simulink model "DynMatProps"  (R2015a)
settings: Solver=FixedStepDiscrete  StartTime=0.0  StopTime=tsim  FixedStep=dt  RelTol=1e-3
values from neighbouring files (symbols this model uses):
  Cp_data = [4.8261 5.46958 6.4348 6.981758 7.56089 8.0435 8.68698]    [run_DynMatProps.m]
  hb = 0.05    [run_DynMatProps.m]
  hl = 0.05    [run_DynMatProps.m]
  hr = 0.05    [run_DynMatProps.m]
  ht = 0.05    [run_DynMatProps.m]
  k_data = [0.013888889 0.016388889 0.020277778 0.022222222 0.027777778 0.029166667 0.027777778]    [run_DynMatProps.m]
  m = length(y0)    [run_DynMatProps.m]
  n = length(x)    [run_DynMatProps.m]
  rho2d = rho*ones(length(y0),length(x))    [run_DynMatProps.m]
  T02d = [T02d T01d']    [run_DynMatProps.m]
  Tb = 1000    [run_DynMatProps.m]
  TCp_data = [259.7 359.7 559.7 659.7 859.7 1059.7 1259.7]    [run_DynMatProps.m]
  Tk_data = [259.7 359.7 559.7 659.7 859.7 1059.7 1259.7]    [run_DynMatProps.m]
  Tl = 1000    [run_DynMatProps.m]
  Tr = 1000    [run_DynMatProps.m]
  Tt = 1000    [run_DynMatProps.m]
libraries: lib_Conduction_2DCondFullyImplicit x1
settings Model: Creator=jlkratz  LastModifiedBy=jlkratz

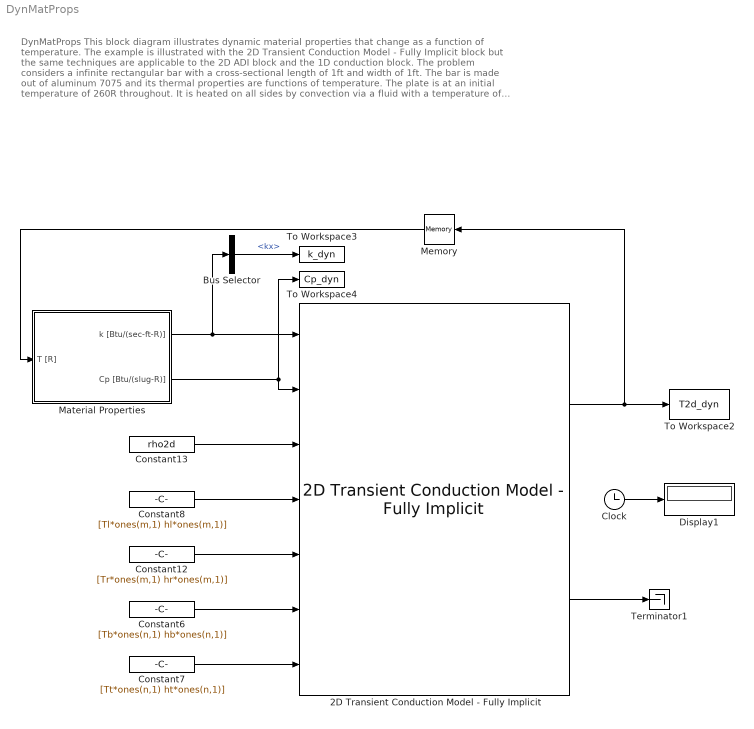
== system DynMatProps ==
  note: DynMatProps
      |
      | This block diagram illustrates dynamic material properties that change as a function of temperature. The example is
      | illustrated with the 2D Transient Conduction Model - Fully Implicit block but the same techniques are applicable
      | to the 2D ADI block and the 1D conduction block.
      |
      | The problem considers a infinite rectangular bar with a cross-sectional length of 1ft and width of 1ft. The bar is made
      | out of aluminum 7075 and its thermal properties are functions of temperature. The plate is at an initial temperature of
      | 260R throughout. It is heated on all sides by convection via a fluid with a temperature of 1000R and a heat transfer
      | coefficient of 0.05Btu/(sec-ft^2-R)
  2D Transient Conduction Model - Fully Implicit : lib_Conduction_2DCondFullyImplicit/2D Transient Conduction Model - Fully Implicit  T0_M=T02d  dt_M=dt  x_M=x  y_M=y0  shape_M=Planar in both directions  convL_M=on  radL_M=off  condL_M=off  convR_M=on  radR_M=off  condR_M=off  convB_M=on  radB_M=off  condB_M=off  convT_M=on  radT_M=off  condT_M=off  BN_M=double(gcb)
  Bus Selector : BusSelector  OutputSignals=kx
  Clock : Clock
  Constant12 : Constant  Value=[Tr*ones(m,1) hr*ones(m,1)]
  Constant13 : Constant  Value=rho2d
  Constant6 : Constant  Value=[Tb*ones(n,1) hb*ones(n,1)]
  Constant7 : Constant  Value=[Tt*ones(n,1) ht*ones(n,1)]
  Constant8 : Constant  Value=[Tl*ones(m,1) hl*ones(m,1)]
  Display1 : Display
  Material Properties : Subsystem
  Memory : Memory  X0=T02d
  Terminator1 : Terminator
  To Workspace2 : ToWorkspace  VariableName=T2d_dyn  SaveFormat=Timeseries  SampleTime=-1
  To Workspace3 : ToWorkspace  VariableName=k_dyn  SaveFormat=Timeseries  SampleTime=-1
  To Workspace4 : ToWorkspace  VariableName=Cp_dyn  SaveFormat=Timeseries  SampleTime=-1
  wires:
  Clock/1 -> Display1/1
  Constant7/1 -> 2D Transient Conduction Model - Fully Implicit/7
  Constant8/1 -> 2D Transient Conduction Model - Fully Implicit/4
  Constant12/1 -> 2D Transient Conduction Model - Fully Implicit/5
  Constant13/1 -> 2D Transient Conduction Model - Fully Implicit/3
  2D Transient Conduction Model - Fully Implicit/1 -> Memory/1, To Workspace2/1
  2D Transient Conduction Model - Fully Implicit/2 -> Terminator1/1
  Memory/1 -> Material Properties/1(T [R])
  Material Properties/1(k [Btu/(sec-ft-R)]) -> 2D Transient Conduction Model - Fully Implicit/1, Bus Selector/1
  Material Properties/2(Cp [Btu/(slug-R)]) -> 2D Transient Conduction Model - Fully Implicit/2, To Workspace4/1
  Constant6/1 -> 2D Transient Conduction Model - Fully Implicit/6
  Bus Selector/1 -> To Workspace3/1  "<kx>"

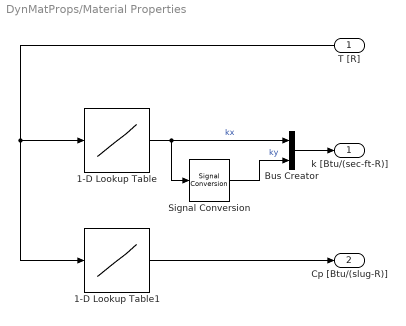
== system DynMatProps/Material Properties ==
  T [R] : Inport
  1-D Lookup Table : Lookup_n-D  NumberOfTableDimensions=1  BreakpointsForDimension1=Tk_data  Table=k_data  InternalRulePriority=Speed  RndMeth=Simplest  InputSameDT=on
  1-D Lookup Table1 : Lookup_n-D  NumberOfTableDimensions=1  BreakpointsForDimension1=TCp_data  Table=Cp_data  InternalRulePriority=Speed  RndMeth=Simplest  InputSameDT=on
  Bus Creator : BusCreator  Inputs=2
  Signal Conversion : SignalConversion
  k [Btu/(sec-ft-R)] : Outport
  Cp [Btu/(slug-R)] : Outport  Port=2
  wires:
  T [R]/1 -> 1-D Lookup Table1/1, 1-D Lookup Table/1
  1-D Lookup Table1/1 -> Cp [Btu/(slug-R)]/1
  Bus Creator/1 -> k [Btu/(sec-ft-R)]/1
  1-D Lookup Table/1 -> Signal Conversion/1, Bus Creator/1  "kx"
  Signal Conversion/1 -> Bus Creator/2  "ky"
